simulink model "caes_extraction"  (R2026a)
settings: Solver=VariableStepAuto
settings Model: Creator=milenadaniltsenko  LastModifiedBy=milenadaniltsenko

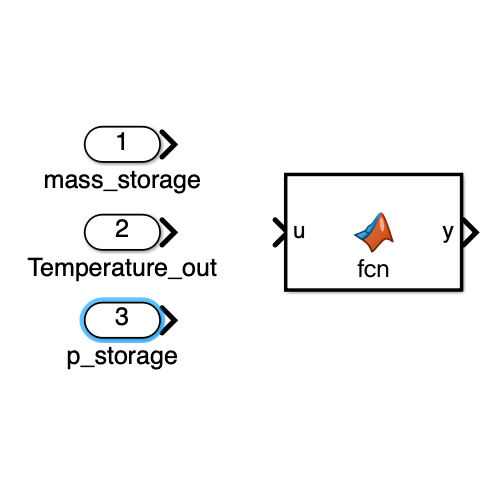
[thumbnail: Simulink's stored preview of the top-level diagram]
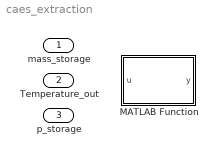
== system caes_extraction ==
  mass_storage : Inport
  Temperature_out : Inport  Port=2
  p_storage : Inport  Port=3
  MATLAB Function : MATLAB Function  TreatAsAtomicUnit=on

== matlab function caes_extraction/MATLAB Function ==
  data: u input; y output
function y = fcn(u)

y = u;
